simulink model "MPSLab1Oles"  (R2014b)
settings: Solver=ode45  StartTime=0.0  StopTime=50  RelTol=1e-3
undefined symbols (not defined in the file): magnitude
settings Model: Creator=kiril_000  LastModifiedBy=kiril_000

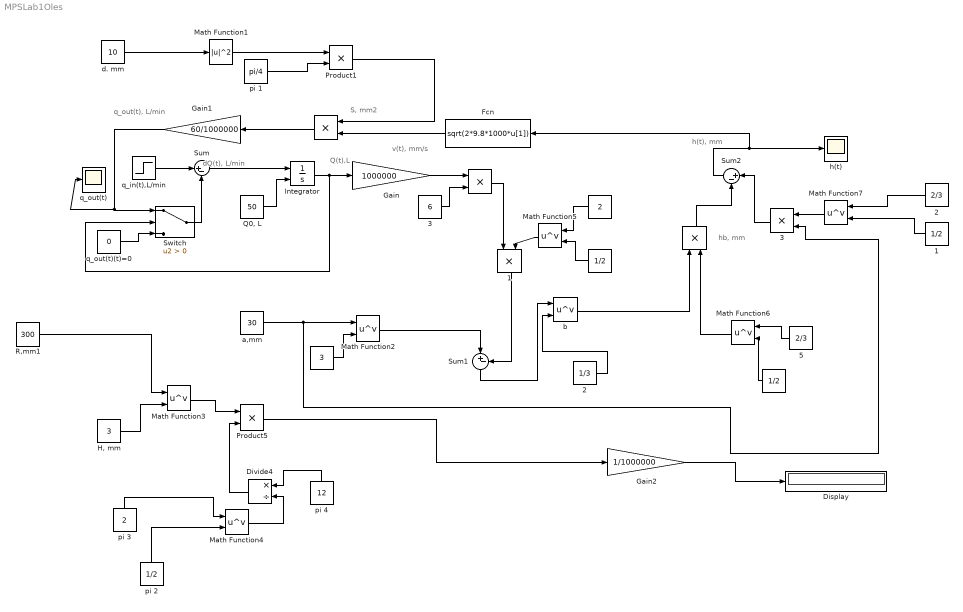
== system MPSLab1Oles ==
  note: h(t), mm
  note: hb, mm
  note: v(t), mm/s
  note: q_out(t), L/min
  note: S, mm2
  note: Q(t),L
  note: dQ(t), L/min
  " " : Constant  Value=1/2
  " 1" : Constant  Value=1/2
  " 2" : Constant  Value=2/3
  " 5" : Constant  Value=2/3
  " " : Constant  Value=2
  " " : Product
  "  " : Product
  " " : Constant  Value=3
  "   " : Product
  "                  " : Constant  Value=1/2
  "  1" : Product
  "  3" : Product
  2 : Constant  Value=1/3
  3 : Constant  Value=6
  Display : Display
  Divide4 : Product  Inputs=*/
  Fcn : Fcn  Expr=sqrt(2*9.8*1000*u[1])
  Gain : Gain  Gain=1000000
  Gain1 : Gain  Gain=60/1000000
  Gain2 : Gain  Gain=1/1000000
  "H, mm" : Constant  Value=3
  Integrator : Integrator  InitialConditionSource=external
  Math Function1 : Math  Operator=magnitude^2  SaturateOnIntegerOverflow=on
  Math Function{2..7} (6 alike) : Math  Operator=pow  SaturateOnIntegerOverflow=on
  Product1 : Product
  Product5 : Product
  "Q0, L" : Constant  Value=50
  R,mm1 : Constant  Value=300
  Sum : Sum  Inputs=|+-
  Sum1 : Sum  Inputs=|+-
  Sum2 : Sum  Inputs=|+-
  Switch : Switch  Criteria=u2 > Threshold
  "a,mm " : Constant  Value=30
  "b " : Math  Operator=pow  SaturateOnIntegerOverflow=on
  d. mm : Constant  Value=10
  h(t) : Scope
      settings: TimeRange=30  YMin=-100  YMax=600
  pi 1 : Constant  Value=pi/4
  pi 2 : Constant  Value=1/2
  pi 3 : Constant  Value=2
  pi 4 : Constant  Value=12
  q_in(t),L/min : Step  Time=10  After=12  SampleTime=0
  q_out(t) : Scope
  q_out(t)(t)=0 : Constant  Value=0
  wires:
  q_in(t),L/min/1 -> Sum/1
  q_out(t)(t)=0/1 -> Switch/3
  Sum/1 -> Integrator/1
  "Q0, L"/1 -> Integrator/2
  Switch/1 -> Sum/2
  Integrator/1 -> Switch/2, Gain/1
  d. mm/1 -> Math Function1/1
  Math Function1/1 -> Product1/1
  pi 1/1 -> Product1/2
  Product1/1 -> "   "/1
  "   "/1 -> Gain1/1
  Fcn/1 -> "   "/2
  3/1 -> " "/2
  Gain/1 -> " "/1
  " "/1 -> "  1"/1
  R,mm1/1 -> Math Function3/1
  Math Function3/1 -> Product5/1
  "H, mm"/1 -> Math Function3/2
  Gain2/1 -> Display/1
  "b "/1 -> "  "/1
  Gain1/1 -> Switch/1, q_out(t)/1
  Math Function5/1 -> "  1"/2
  2/1 -> "b "/2
  pi 2/1 -> Math Function4/2
  pi 3/1 -> Math Function4/1
  Math Function4/1 -> Divide4/2
  Divide4/1 -> Product5/2
  pi 4/1 -> Divide4/1
  " "/1 -> Math Function5/1
  "                  "/1 -> Math Function5/2
  " 5"/1 -> Math Function6/1
  " "/1 -> Math Function6/2
  Math Function6/1 -> "  "/2
  Product5/1 -> Gain2/1
  "a,mm "/1 -> "  3"/2, Math Function2/1
  " "/1 -> Math Function2/2
  Math Function2/1 -> Sum1/1
  "  1"/1 -> Sum1/2
  Sum1/1 -> "b "/1
  " 2"/1 -> Math Function7/1
  " 1"/1 -> Math Function7/2
  Math Function7/1 -> "  3"/1
  "  "/1 -> Sum2/2
  "  3"/1 -> Sum2/1
  Sum2/1 -> Fcn/1, h(t)/1
